simulink model "Test"  (R2019b)
settings: Solver=VariableStepAuto  StartTime=0.0  StopTime=10.0  RelTol=1e-3
settings Model: Creator=bsu  LastModifiedBy=bsu

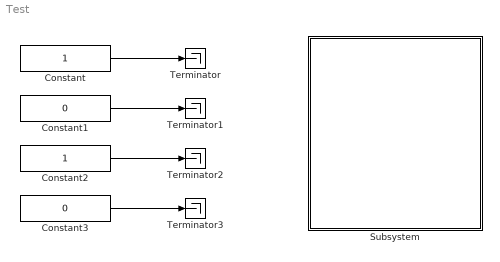
== system Test ==
  Constant : Constant
  Constant1 : Constant  Value=0
  Constant2 : Constant
  Constant3 : Constant  Value=0
  Subsystem : Subsystem
  Terminator{,1..3} (4 alike) : Terminator
  wires:
  Constant/1 -> Terminator/1
  Constant1/1 -> Terminator1/1
  Constant2/1 -> Terminator2/1
  Constant3/1 -> Terminator3/1

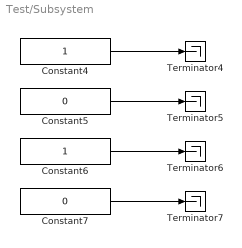
== system Test/Subsystem ==
  Constant4 : Constant
  Constant5 : Constant  Value=0
  Constant6 : Constant
  Constant7 : Constant  Value=0
  Terminator{4..7} (4 alike) : Terminator
  wires:
  Constant6/1 -> Terminator6/1
  Constant7/1 -> Terminator7/1
  Constant4/1 -> Terminator4/1
  Constant5/1 -> Terminator5/1
